simulink model "method4"  (R2025a)
settings: Solver=ode45  StartTime=0.0  StopTime=100  FixedStep=0.01  MaxStep=0.001  RelTol=1e-3
settings Model: Creator=vm66c  LastModifiedBy=vm66c
settings DataIOCC: ReturnWorkspaceOutputs=off

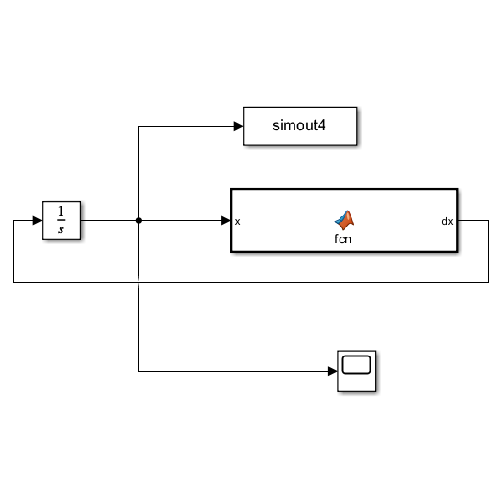
[thumbnail: Simulink's stored preview of the top-level diagram]
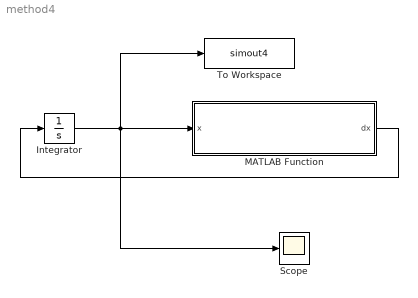
== system method4 ==
  Integrator : Integrator  InitialCondition=[0, 0, 1e-10]'
  MATLAB Function : MATLAB Function  TreatAsAtomicUnit=on
  Scope : Scope
      settings: ActiveDisplayYMinimum=-23.956687842456084  ActiveDisplayYMaximum=52.5163554630408
  To Workspace : ToWorkspace  VariableName=simout4  SampleTime=-1
  wires:
  Integrator/1 -> To Workspace/1, Scope/1, MATLAB Function/1(x)
  MATLAB Function/1(dx) -> Integrator/1

== matlab function method4/MATLAB Function ==
  data: x input; dx output
function dx = fcn(x)
    % 输入 x 是一个 3x1 的向量 [x1; x2; x3]
    % 严格按照作业要求的公式编写
    dx = zeros(3,1);
    
    dx(1) = -8/3 * x(1) + x(2) * x(3);        % 对应方程 1
    dx(2) = -10 * x(2) + 10 * x(3);           % 对应方程 2
    dx(3) = -x(1) * x(2) + 28 * x(2) - x(3);  % 对应方程 3
end
